simulink model "mass_spring_damper_simulink"  (R2024b)
settings: Solver=VariableStepAuto  StartTime=0.0  StopTime=Sim_Time  RelTol=1e-3
undefined symbols (not defined in the file): b, k, M
settings Model: Creator=Lenovo  LastModifiedBy=Lenovo

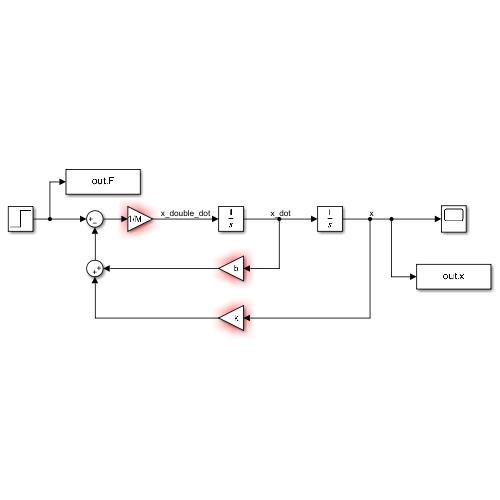
[thumbnail: Simulink's stored preview of the top-level diagram]
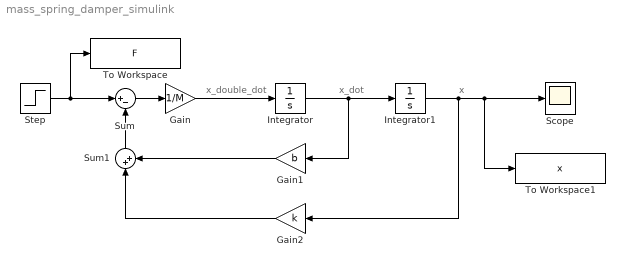
== system mass_spring_damper_simulink ==
  note: x_double_dot
  note: x_dot
  note: x
  Gain : Gain  Gain=1/M
  Gain1 : Gain  Gain=b
  Gain2 : Gain  Gain=k
  Integrator : Integrator
  Integrator1 : Integrator
  Scope : Scope
  Step : Step  SampleTime=0
  Sum : Sum  Inputs=|+-
  Sum1 : Sum  Inputs=|++
  To Workspace : ToWorkspace  VariableName=F  SaveFormat=Timeseries  SampleTime=-1
  To Workspace1 : ToWorkspace  VariableName=x  SaveFormat=Timeseries  SampleTime=-1
  wires:
  Integrator/1 -> Gain1/1, Integrator1/1
  Gain/1 -> Integrator/1
  Integrator1/1 -> To Workspace1/1, Scope/1, Gain2/1
  Sum1/1 -> Sum/2
  Step/1 -> To Workspace/1, Sum/1
  Sum/1 -> Gain/1
  Gain1/1 -> Sum1/2
  Gain2/1 -> Sum1/1
